simulink model "ES105A_StHlthSigNormn"  (R2013b)
settings: Solver=FixedStepDiscrete  SolverMode=SingleTasking  StartTime=0.0  StopTime=1  FixedStep=0.002  RelTol=1e-3
undefined symbols (not defined in the file): ARCHGLBPRM_FLOATZEROTHD_ULS_F32, CurrMeasCorrlnMaxErrCurr, CURRMOTSUMDIVBYZEROPROTNVAL_AMPR_F32, DIGTQDIVBYZEROPROTNVAL_HWNWTMTR_F32, DutyCycThermProtnDutyCycFildThd, EcuTMeasRngDiagcMax, EcuTMeasRngDiagcMin, EotLrngAuthyStrtLrn, FRICESTIMNDIVBYZEROPROTNVAL_HWNWTMTR_F32, HLTH0PERC_CNT_U08, HLTH100PERC_CNT_F32, HLTH100PERC_CNT_U08, HLTH50PERC_CNT_U08, HwTqCorrlnChATraSumSetFltThd, HwTqCorrlnChBTraSumSetFltThd, HWTQIDPTSIG_CNT_U08, MOTAG2MEAS_VALMAXERR_VOLTSQD_F32, MOTAG2MEAS_VALMINERR_VOLTSQD_F32, MOTAGCORRLN_MOTAGCORRLNERRTHD_MOTREVELEC_U0P16, MotDrvDiagcErrThd, MOTPOS2DIVBYZEROPROTNVAL2_VOLTSQD_F32, MOTPOS2DIVBYZEROPROTNVAL_VOLTSQD_F32, MOTPOSNERRDIVBYZEROPROTNVAL_MOTREV_U16, MOTPOSNERRZEROTHD_MOTREV_U0P16, NtcNr1, NtcSts1, PHAVLTGDIVBYZEROPROTNVAL_NANOSEC_F32, SigQlfr1, STHLTHSCAGFAC_CNT_F32, StHlthSigNormnAbsltMotPosDifStHlthDiagThd, StHlthSigNormnCurrMotSumStHlthDiagThd, StHlthSigNormnDigTqStHlthDiagThd, StHlthSigNormnDutyCycFltLimThd, StHlthSigNormnHiCtrlrT, StHlthSigNormnIdptSigStHlthSca, StHlthSigNormnLoCtrlrT, StHlthSigNormnMaxFricThd, StHlthSigNormnMinRackTrvlLim, StHlthSigNormnMotPosStHlthDiagThd, StHlthSigNormnMotVelCal, StHlthSigNormnPhaInfoStHlthDiagThd, StHlthSigNormnStHlthCorrlnErr, StHlthSigNormnStHlthCurrMotSum, StHlthSigNormnStHlthPhaInfo, StHlthSigNormnValMaxStHlthErr, StHlthSigNormnValMinStHlthErr, StHlthSigNormnWhlImbRejctnThd, SysGlbPrmMotPoleCnt, TSTHLTH0PERC_CNT_U08, u2, u3, u4, VLTGSTHLTH0PERC_CNT_U08
libraries: NxtrLim x39, simulink x33, NxtrAbslt x4
(part 6 of 10)

== system ES105A_StHlthSigNormn/StHlthSigNormn/UpdRawSig/Digital Torque Sensor /DigTqSnsrAStHlth Calc/If Action Subsystem1 ==
  HwTqChACorrlnTraErr : Inport
  Action Port : ActionPort  ActionType=else
  Abslt_f32_f32 : NxtrAbslt/Abslt_f32_f32  SFunctionSpec=single y1 = Abslt_f32_f32(single u1)
      settings: AttributesFormatString=%<Name>
  Constant2 : Constant  OutDataTypeStr=single
      settings: AttributesFormatString=%<OutDataTypeStr>
  Constant3 : Constant  Value=STHLTHSCAGFAC_CNT_F32
  CopyRight2 : Subsystem  Description=|  mask(Copyright Information){none=on}
      | Copyright info block.                                               
      |                                                                     
      | Place copyright information at the top of every subsystem in design.
      mask prompts: none "No parameters"
      mask help: Place copyright information at the top of every subsystem in design.
      mask Display:
      | NxtrConf = 'Nexteer Confidential';
      | 
      | sys = bdroot; %handle for the current model ("system")
      | first = get_param(sys,'Created');
      | first = first(end-3:end);  %year is last four digits
      | 
      | last = get_param(sys,'LastModifiedDate');
      | if isempty(last)
      |     last = datestr(now,'yyyy');
      | else
      |     last = last(end-3:end);
      | end
      | 
      | if strcmp(first,last)
      |     fprintf('%s -- Copyright %s Nexteer',NxtrConf,first)
      | else
      |     fprintf('%s -- %s%s- %s Nexteer',NxtrConf,char(169),first,last)
      | end
  Data Type Conversion : DataTypeConversion  OutDataTypeStr=uint8
  Devide by Zero Protection for Cal : Subsystem
  Divide : Product  Inputs=*/
  LimStat_f32 : NxtrLim/LimStat_f32  LoLim=STHLTHFLOATZEROVAL_ULS_F32  HiLim=STHLTHFLOATTWOFIFTYFIVEVAL_ULS_F32
      settings: AttributesFormatString=|
      | Low Limit: %<LoLim>
      | High Limit:%<HiLim>
  Product : Product
  Subtract : Sum  Inputs=+-
  DigTqSnsrAStHlth : Outport
  wires:
  HwTqChACorrlnTraErr/1 -> Divide/1
  Divide/1 -> Abslt_f32_f32/1
  Abslt_f32_f32/1 -> Subtract/2
  Constant2/1 -> Subtract/1
  Constant3/1 -> Product/2
  Data Type Conversion/1 -> DigTqSnsrAStHlth/1
  Subtract/1 -> Product/1
  Devide by Zero Protection for Cal/1(HwTqCorrlnChATraSumSetFltThd) -> Divide/2
  LimStat_f32/1 -> Data Type Conversion/1
  Product/1 -> LimStat_f32/1

== system ES105A_StHlthSigNormn/StHlthSigNormn/UpdRawSig/Digital Torque Sensor /DigTqSnsrBStHlth Calc/CopyRight2 ==

== system ES105A_StHlthSigNormn/StHlthSigNormn/UpdRawSig/Digital Torque Sensor /DigTqSnsrBStHlth Calc/If Action Subsystem2 ==
  Action Port : ActionPort  ActionType=then
  Constant : Constant  Value=HLTH0PERC_CNT_U08  OutDataTypeStr=uint8
  CopyRight2 : Subsystem  Description=|  mask(Copyright Information){none=on}
      | Copyright info block.                                               
      |                                                                     
      | Place copyright information at the top of every subsystem in design.
      mask prompts: none "No parameters"
      mask help: Place copyright information at the top of every subsystem in design.
      mask Display:
      | NxtrConf = 'Nexteer Confidential';
      | 
      | sys = bdroot; %handle for the current model ("system")
      | first = get_param(sys,'Created');
      | first = first(end-3:end);  %year is last four digits
      | 
      | last = get_param(sys,'LastModifiedDate');
      | if isempty(last)
      |     last = datestr(now,'yyyy');
      | else
      |     last = last(end-3:end);
      | end
      | 
      | if strcmp(first,last)
      |     fprintf('%s -- Copyright %s Nexteer',NxtrConf,first)
      | else
      |     fprintf('%s -- %s%s- %s Nexteer',NxtrConf,char(169),first,last)
      | end
  DigTqSnsrBStHlth : Outport
  wires:
  Constant/1 -> DigTqSnsrBStHlth/1

== system ES105A_StHlthSigNormn/StHlthSigNormn/UpdRawSig/Digital Torque Sensor /DigTqSnsrBStHlth Calc/If Action Subsystem3 ==
  HwTqChBCorrlnTraErr : Inport
  Action Port : ActionPort  ActionType=else
  Abslt_f32_f32 : NxtrAbslt/Abslt_f32_f32  SFunctionSpec=single y1 = Abslt_f32_f32(single u1)
      settings: AttributesFormatString=%<Name>
  Constant2 : Constant  OutDataTypeStr=single
      settings: AttributesFormatString=%<OutDataTypeStr>
  Constant3 : Constant  Value=STHLTHSCAGFAC_CNT_F32
  CopyRight2 : Subsystem  Description=|  mask(Copyright Information){none=on}
      | Copyright info block.                                               
      |                                                                     
      | Place copyright information at the top of every subsystem in design.
      mask prompts: none "No parameters"
      mask help: Place copyright information at the top of every subsystem in design.
      mask Display:
      | NxtrConf = 'Nexteer Confidential';
      | 
      | sys = bdroot; %handle for the current model ("system")
      | first = get_param(sys,'Created');
      | first = first(end-3:end);  %year is last four digits
      | 
      | last = get_param(sys,'LastModifiedDate');
      | if isempty(last)
      |     last = datestr(now,'yyyy');
      | else
      |     last = last(end-3:end);
      | end
      | 
      | if strcmp(first,last)
      |     fprintf('%s -- Copyright %s Nexteer',NxtrConf,first)
      | else
      |     fprintf('%s -- %s%s- %s Nexteer',NxtrConf,char(169),first,last)
      | end
  Data Type Conversion : DataTypeConversion  OutDataTypeStr=uint8
  Devide by Zero Protection for Cal : Subsystem
  Divide : Product  Inputs=*/
  LimStat_f32 : NxtrLim/LimStat_f32  LoLim=STHLTHFLOATZEROVAL_ULS_F32  HiLim=STHLTHFLOATTWOFIFTYFIVEVAL_ULS_F32
      settings: AttributesFormatString=|
      | Low Limit: %<LoLim>
      | High Limit:%<HiLim>
  Product : Product
  Subtract : Sum  Inputs=+-
  DigTqSnsrBStHlth : Outport
  wires:
  HwTqChBCorrlnTraErr/1 -> Divide/1
  Divide/1 -> Abslt_f32_f32/1
  Abslt_f32_f32/1 -> Subtract/2
  Constant2/1 -> Subtract/1
  Constant3/1 -> Product/2
  Subtract/1 -> Product/1
  Devide by Zero Protection for Cal/1(HwTqCorrlnChBTraSumSetFltThd) -> Divide/2
  LimStat_f32/1 -> Data Type Conversion/1
  Product/1 -> LimStat_f32/1
  Data Type Conversion/1 -> DigTqSnsrBStHlth/1

== system ES105A_StHlthSigNormn/StHlthSigNormn/UpdRawSig/Digital Torque Sensor /DigTqSnsrPhaStHlth/SetNtcSts ==
  note: Note:
      |
      | - "ISO Fault Debounce Design" Simulink block intent to use here for Simulation purpose only. Do not Code this block
  NtcNr : Inport
  NtcStInfo : Inport  Port=2
  NtcSts : Inport  Port=3
  DebStep : Inport  Port=4
  CopyRight2 : Subsystem  Description=|  mask(Copyright Information){none=on}
      | Copyright info block.                                               
      |                                                                     
      | Place copyright information at the top of every subsystem in design.
      mask prompts: none "No parameters"
      mask help: Place copyright information at the top of every subsystem in design.
      mask Display:
      | NxtrConf = 'Nexteer Confidential';
      | 
      | sys = bdroot; %handle for the current model ("system")
      | first = get_param(sys,'Created');
      | first = first(end-3:end);  %year is last four digits
      | 
      | last = get_param(sys,'LastModifiedDate');
      | if isempty(last)
      |     last = datestr(now,'yyyy');
      | else
      |     last = last(end-3:end);
      | end
      | 
      | if strcmp(first,last)
      |     fprintf('%s -- Copyright %s Nexteer',NxtrConf,first)
      | else
      |     fprintf('%s -- %s%s- %s Nexteer',NxtrConf,char(169),first,last)
      | end
  Data Store Write : DataStoreWrite  DataStoreName=NtcQlfr0X1D0
  Ground : Ground
  ISO Fault Debounce Design : Stateflow chart  TreatAsAtomicUnit=on
      settings: AttributesFormatString=|
      | Simulation Purpose Only.
      | Do Not Code this block
      | Diagnostic Manager Owns this requirement
  Terminator : Terminator
  Terminator1 : Terminator
  wires:
  NtcStInfo/1 -> Terminator1/1
  NtcNr/1 -> Terminator/1
  NtcSts/1 -> ISO Fault Debounce Design/1(NtcSts)
  DebStep/1 -> ISO Fault Debounce Design/2(DebStep)
  ISO Fault Debounce Design/1(Qualifier) -> Data Store Write/1
  Ground/1 -> ISO Fault Debounce Design/3(SvcClr)

== system ES105A_StHlthSigNormn/StHlthSigNormn/UpdRawSig/Digital Torque Sensor /NTC Sts Calculation/CopyRight2 ==

== system ES105A_StHlthSigNormn/StHlthSigNormn/UpdRawSig/Digital Torque Sensor /NTC Sts Calculation/NtcFaild ==
  Action Port : ActionPort  ActionType=then
  Constant2 : Constant  Value=NtcSts1.NTCSTS_FAILD  OutDataTypeStr=Enum: NtcSts1
  CopyRight2 : Subsystem  Description=|  mask(Copyright Information){none=on}
      | Copyright info block.                                               
      |                                                                     
      | Place copyright information at the top of every subsystem in design.
      mask prompts: none "No parameters"
      mask help: Place copyright information at the top of every subsystem in design.
      mask Display:
      | NxtrConf = 'Nexteer Confidential';
      | 
      | sys = bdroot; %handle for the current model ("system")
      | first = get_param(sys,'Created');
      | first = first(end-3:end);  %year is last four digits
      | 
      | last = get_param(sys,'LastModifiedDate');
      | if isempty(last)
      |     last = datestr(now,'yyyy');
      | else
      |     last = last(end-3:end);
      | end
      | 
      | if strcmp(first,last)
      |     fprintf('%s -- Copyright %s Nexteer',NxtrConf,first)
      | else
      |     fprintf('%s -- %s%s- %s Nexteer',NxtrConf,char(169),first,last)
      | end
  NtcFaild : Outport
  wires:
  Constant2/1 -> NtcFaild/1

== system ES105A_StHlthSigNormn/StHlthSigNormn/UpdRawSig/Digital Torque Sensor /NTC Sts Calculation/NtcPassd ==
  Action Port : ActionPort  ActionType=else
  Constant2 : Constant  Value=NtcSts1.NTCSTS_PASSD  OutDataTypeStr=Enum: NtcSts1
  CopyRight2 : Subsystem  Description=|  mask(Copyright Information){none=on}
      | Copyright info block.                                               
      |                                                                     
      | Place copyright information at the top of every subsystem in design.
      mask prompts: none "No parameters"
      mask help: Place copyright information at the top of every subsystem in design.
      mask Display:
      | NxtrConf = 'Nexteer Confidential';
      | 
      | sys = bdroot; %handle for the current model ("system")
      | first = get_param(sys,'Created');
      | first = first(end-3:end);  %year is last four digits
      | 
      | last = get_param(sys,'LastModifiedDate');
      | if isempty(last)
      |     last = datestr(now,'yyyy');
      | else
      |     last = last(end-3:end);
      | end
      | 
      | if strcmp(first,last)
      |     fprintf('%s -- Copyright %s Nexteer',NxtrConf,first)
      | else
      |     fprintf('%s -- %s%s- %s Nexteer',NxtrConf,char(169),first,last)
      | end
  NtcPassd : Outport
  wires:
  Constant2/1 -> NtcPassd/1

== system ES105A_StHlthSigNormn/StHlthSigNormn/UpdRawSig/Duty Cycle Exceeded/If Action Subsystem/CopyRight2 ==

== system ES105A_StHlthSigNormn/StHlthSigNormn/UpdRawSig/Duty Cycle Exceeded/If Action Subsystem1/CopyRight2 ==

== system ES105A_StHlthSigNormn/StHlthSigNormn/UpdRawSig/Duty Cycle Exceeded/If Action Subsystem2/CopyRight2 ==

== system ES105A_StHlthSigNormn/StHlthSigNormn/UpdRawSig/Friction Estimation/If Action Subsystem3/CopyRight2 ==

== system ES105A_StHlthSigNormn/StHlthSigNormn/UpdRawSig/Friction Estimation/If Action Subsystem4/CopyRight2 ==

== system ES105A_StHlthSigNormn/StHlthSigNormn/UpdRawSig/Friction Estimation/If Action Subsystem4/Divide by Zero Protection for Cal ==
  EOLFric : Inport
  Add1 : Sum  Inputs=+-
  Constant : Constant  Value=ARCHGLBPRM_FLOATZEROTHD_ULS_F32
  Constant2 : Constant  Value=StHlthSigNormnMaxFricThd
  CopyRight2 : Subsystem  Description=|  mask(Copyright Information){none=on}
      | Copyright info block.                                               
      |                                                                     
      | Place copyright information at the top of every subsystem in design.
      mask prompts: none "No parameters"
      mask help: Place copyright information at the top of every subsystem in design.
      mask Display:
      | NxtrConf = 'Nexteer Confidential';
      | 
      | sys = bdroot; %handle for the current model ("system")
      | first = get_param(sys,'Created');
      | first = first(end-3:end);  %year is last four digits
      | 
      | last = get_param(sys,'LastModifiedDate');
      | if isempty(last)
      |     last = datestr(now,'yyyy');
      | else
      |     last = last(end-3:end);
      | end
      | 
      | if strcmp(first,last)
      |     fprintf('%s -- Copyright %s Nexteer',NxtrConf,first)
      | else
      |     fprintf('%s -- %s%s- %s Nexteer',NxtrConf,char(169),first,last)
      | end
  If : If  IfExpression=u1
  If Zero : Subsystem  TreatAsAtomicUnit=on
  Merge : Merge
  Non Zero : Subsystem  TreatAsAtomicUnit=on
  Relational Operator : RelationalOperator  Operator=<=  OutDataTypeStr=boolean
  FricEstDelta : Outport
  wires:
  If/1 -> If Zero/Action
  If/2 -> Non Zero/Action
  If Zero/1(Out1) -> Merge/1
  Non Zero/1(Out1) -> Merge/2
  Merge/1 -> FricEstDelta/1
  Relational Operator/1 -> If/1
  Constant/1 -> Relational Operator/2
  Constant2/1 -> Add1/1
  EOLFric/1 -> Add1/2
  Add1/1 -> Non Zero/1(In1), Relational Operator/1

== system ES105A_StHlthSigNormn/StHlthSigNormn/UpdRawSig/Motor Position 2 /If Action Subsystem/CopyRight2 ==

== system ES105A_StHlthSigNormn/StHlthSigNormn/UpdRawSig/Motor Position 2 /If Action Subsystem/If Action Subsystem ==
  Action Port : ActionPort  ActionType=then
  Constant : Constant  Value=HLTH0PERC_CNT_U08
  CopyRight2 : Subsystem  Description=|  mask(Copyright Information){none=on}
      | Copyright info block.                                               
      |                                                                     
      | Place copyright information at the top of every subsystem in design.
      mask prompts: none "No parameters"
      mask help: Place copyright information at the top of every subsystem in design.
      mask Display:
      | NxtrConf = 'Nexteer Confidential';
      | 
      | sys = bdroot; %handle for the current model ("system")
      | first = get_param(sys,'Created');
      | first = first(end-3:end);  %year is last four digits
      | 
      | last = get_param(sys,'LastModifiedDate');
      | if isempty(last)
      |     last = datestr(now,'yyyy');
      | else
      |     last = last(end-3:end);
      | end
      | 
      | if strcmp(first,last)
      |     fprintf('%s -- Copyright %s Nexteer',NxtrConf,first)
      | else
      |     fprintf('%s -- %s%s- %s Nexteer',NxtrConf,char(169),first,last)
      | end
  MotPosStHlth : Outport
  wires:
  Constant/1 -> MotPosStHlth/1

== system ES105A_StHlthSigNormn/StHlthSigNormn/UpdRawSig/Motor Position 2 /If Action Subsystem/If Action Subsystem1 ==
  MotAg2VltgSqd : Inport
  Action Port : ActionPort  ActionType=elseif
  Constant : Constant  Value=MOTAG2MEAS_VALMINERR_VOLTSQD_F32
  Constant3 : Constant  Value=STHLTHSCAGFAC_CNT_F32
  CopyRight2 : Subsystem  Description=|  mask(Copyright Information){none=on}
      | Copyright info block.                                               
      |                                                                     
      | Place copyright information at the top of every subsystem in design.
      mask prompts: none "No parameters"
      mask help: Place copyright information at the top of every subsystem in design.
      mask Display:
      | NxtrConf = 'Nexteer Confidential';
      | 
      | sys = bdroot; %handle for the current model ("system")
      | first = get_param(sys,'Created');
      | first = first(end-3:end);  %year is last four digits
      | 
      | last = get_param(sys,'LastModifiedDate');
      | if isempty(last)
      |     last = datestr(now,'yyyy');
      | else
      |     last = last(end-3:end);
      | end
      | 
      | if strcmp(first,last)
      |     fprintf('%s -- Copyright %s Nexteer',NxtrConf,first)
      | else
      |     fprintf('%s -- %s%s- %s Nexteer',NxtrConf,char(169),first,last)
      | end
  Data Type Conversion : DataTypeConversion  OutDataTypeStr=uint8
  Divide : Product  Inputs=*/
  Divide by Zero Protection for Cal : Subsystem
  LimStat_f32 : NxtrLim/LimStat_f32  LoLim=STHLTHFLOATZEROVAL_ULS_F32  HiLim=STHLTHFLOATTWOFIFTYFIVEVAL_ULS_F32
      settings: AttributesFormatString=|
      | Low Limit: %<LoLim>
      | High Limit:%<HiLim>
  Product : Product
  Subtract : Sum  Inputs=+-
  MotPosStHlth : Outport
  wires:
  MotAg2VltgSqd/1 -> Subtract/1
  Constant/1 -> Subtract/2
  Subtract/1 -> Divide/1
  Constant3/1 -> Product/2
  Product/1 -> LimStat_f32/1
  Divide/1 -> Product/1
  Divide by Zero Protection for Cal/1(MotorPos2DeltaMin) -> Divide/2
  LimStat_f32/1 -> Data Type Conversion/1
  Data Type Conversion/1 -> MotPosStHlth/1

== system ES105A_StHlthSigNormn/StHlthSigNormn/UpdRawSig/Motor Position 2 /If Action Subsystem/If Action Subsystem2 ==
  MotAg2VltgSqd : Inport
  Action Port : ActionPort  ActionType=else
  Constant1 : Constant  Value=MOTAG2MEAS_VALMAXERR_VOLTSQD_F32
  Constant3 : Constant  Value=STHLTHSCAGFAC_CNT_F32
  CopyRight2 : Subsystem  Description=|  mask(Copyright Information){none=on}
      | Copyright info block.                                               
      |                                                                     
      | Place copyright information at the top of every subsystem in design.
      mask prompts: none "No parameters"
      mask help: Place copyright information at the top of every subsystem in design.
      mask Display:
      | NxtrConf = 'Nexteer Confidential';
      | 
      | sys = bdroot; %handle for the current model ("system")
      | first = get_param(sys,'Created');
      | first = first(end-3:end);  %year is last four digits
      | 
      | last = get_param(sys,'LastModifiedDate');
      | if isempty(last)
      |     last = datestr(now,'yyyy');
      | else
      |     last = last(end-3:end);
      | end
      | 
      | if strcmp(first,last)
      |     fprintf('%s -- Copyright %s Nexteer',NxtrConf,first)
      | else
      |     fprintf('%s -- %s%s- %s Nexteer',NxtrConf,char(169),first,last)
      | end
  Data Type Conversion : DataTypeConversion  OutDataTypeStr=uint8
  Divide : Product  Inputs=*/
  Divide by Zero Protection for Cal : Subsystem
  LimStat_f32 : NxtrLim/LimStat_f32  LoLim=STHLTHFLOATZEROVAL_ULS_F32  HiLim=STHLTHFLOATTWOFIFTYFIVEVAL_ULS_F32
      settings: AttributesFormatString=|
      | Low Limit: %<LoLim>
      | High Limit:%<HiLim>
  Product : Product
  Subtract1 : Sum  Inputs=+-
  MotPosStHlth : Outport
  wires:
  Constant3/1 -> Product/2
  Constant1/1 -> Subtract1/1
  MotAg2VltgSqd/1 -> Subtract1/2
  Subtract1/1 -> Divide/1
  Divide/1 -> Product/1
  Divide by Zero Protection for Cal/1(MotorPos2DeltaMax) -> Divide/2
  Product/1 -> LimStat_f32/1
  LimStat_f32/1 -> Data Type Conversion/1
  Data Type Conversion/1 -> MotPosStHlth/1

== system ES105A_StHlthSigNormn/StHlthSigNormn/UpdRawSig/Motor Position 2 /If Action Subsystem1/CopyRight2 ==

== system ES105A_StHlthSigNormn/StHlthSigNormn/UpdRawSig/Motor Position 2 /NTC Sts Calculation/CopyRight2 ==

== system ES105A_StHlthSigNormn/StHlthSigNormn/UpdRawSig/Motor Position 2 /NTC Sts Calculation/NtcFaild ==
  Action Port : ActionPort  ActionType=then
  Constant2 : Constant  Value=NtcSts1.NTCSTS_FAILD  OutDataTypeStr=Enum: NtcSts1
  CopyRight2 : Subsystem  Description=|  mask(Copyright Information){none=on}
      | Copyright info block.                                               
      |                                                                     
      | Place copyright information at the top of every subsystem in design.
      mask prompts: none "No parameters"
      mask help: Place copyright information at the top of every subsystem in design.
      mask Display:
      | NxtrConf = 'Nexteer Confidential';
      | 
      | sys = bdroot; %handle for the current model ("system")
      | first = get_param(sys,'Created');
      | first = first(end-3:end);  %year is last four digits
      | 
      | last = get_param(sys,'LastModifiedDate');
      | if isempty(last)
      |     last = datestr(now,'yyyy');
      | else
      |     last = last(end-3:end);
      | end
      | 
      | if strcmp(first,last)
      |     fprintf('%s -- Copyright %s Nexteer',NxtrConf,first)
      | else
      |     fprintf('%s -- %s%s- %s Nexteer',NxtrConf,char(169),first,last)
      | end
  NtcFaild : Outport
  wires:
  Constant2/1 -> NtcFaild/1

== system ES105A_StHlthSigNormn/StHlthSigNormn/UpdRawSig/Motor Position 2 /NTC Sts Calculation/NtcPassd ==
  Action Port : ActionPort  ActionType=else
  Constant2 : Constant  Value=NtcSts1.NTCSTS_PASSD  OutDataTypeStr=Enum: NtcSts1
  CopyRight2 : Subsystem  Description=|  mask(Copyright Information){none=on}
      | Copyright info block.                                               
      |                                                                     
      | Place copyright information at the top of every subsystem in design.
      mask prompts: none "No parameters"
      mask help: Place copyright information at the top of every subsystem in design.
      mask Display:
      | NxtrConf = 'Nexteer Confidential';
      | 
      | sys = bdroot; %handle for the current model ("system")
      | first = get_param(sys,'Created');
      | first = first(end-3:end);  %year is last four digits
      | 
      | last = get_param(sys,'LastModifiedDate');
      | if isempty(last)
      |     last = datestr(now,'yyyy');
      | else
      |     last = last(end-3:end);
      | end
      | 
      | if strcmp(first,last)
      |     fprintf('%s -- Copyright %s Nexteer',NxtrConf,first)
      | else
      |     fprintf('%s -- %s%s- %s Nexteer',NxtrConf,char(169),first,last)
      | end
  NtcPassd : Outport
  wires:
  Constant2/1 -> NtcPassd/1

== system ES105A_StHlthSigNormn/StHlthSigNormn/UpdRawSig/Motor Position 2 /NtcMotPosStHlth/SetNtcSts ==
  note: Note:
      |
      | - "ISO Fault Debounce Design" Simulink block intent to use here for Simulation purpose only. Do not Code this block
  NtcNr : Inport
  NtcStInfo : Inport  Port=2
  NtcSts : Inport  Port=3
  DebStep : Inport  Port=4
  CopyRight2 : Subsystem  Description=|  mask(Copyright Information){none=on}
      | Copyright info block.                                               
      |                                                                     
      | Place copyright information at the top of every subsystem in design.
      mask prompts: none "No parameters"
      mask help: Place copyright information at the top of every subsystem in design.
      mask Display:
      | NxtrConf = 'Nexteer Confidential';
      | 
      | sys = bdroot; %handle for the current model ("system")
      | first = get_param(sys,'Created');
      | first = first(end-3:end);  %year is last four digits
      | 
      | last = get_param(sys,'LastModifiedDate');
      | if isempty(last)
      |     last = datestr(now,'yyyy');
      | else
      |     last = last(end-3:end);
      | end
      | 
      | if strcmp(first,last)
      |     fprintf('%s -- Copyright %s Nexteer',NxtrConf,first)
      | else
      |     fprintf('%s -- %s%s- %s Nexteer',NxtrConf,char(169),first,last)
      | end
  Data Store Write : DataStoreWrite  DataStoreName=NtcQlfr0X1D1
  Ground : Ground
  ISO Fault Debounce Design : Stateflow chart  TreatAsAtomicUnit=on
      settings: AttributesFormatString=|
      | Simulation Purpose Only.
      | Do Not Code this block
      | Diagnostic Manager Owns this requirement
  Terminator : Terminator
  Terminator1 : Terminator
  wires:
  NtcStInfo/1 -> Terminator1/1
  NtcNr/1 -> Terminator/1
  NtcSts/1 -> ISO Fault Debounce Design/1(NtcSts)
  DebStep/1 -> ISO Fault Debounce Design/2(DebStep)
  ISO Fault Debounce Design/1(Qualifier) -> Data Store Write/1
  Ground/1 -> ISO Fault Debounce Design/3(SvcClr)

== system ES105A_StHlthSigNormn/StHlthSigNormn/UpdRawSig/Motor Position Error /AbsltMotPosABDifStHlth Calc/CopyRight2 ==

== system ES105A_StHlthSigNormn/StHlthSigNormn/UpdRawSig/Motor Position Error /AbsltMotPosABDifStHlth Calc/If Action Subsystem ==
  MotAgABErrTerm : Inport
  Action Port : ActionPort  ActionType=then
  CopyRight2 : Subsystem  Description=|  mask(Copyright Information){none=on}
      | Copyright info block.                                               
      |                                                                     
      | Place copyright information at the top of every subsystem in design.
      mask prompts: none "No parameters"
      mask help: Place copyright information at the top of every subsystem in design.
      mask Display:
      | NxtrConf = 'Nexteer Confidential';
      | 
      | sys = bdroot; %handle for the current model ("system")
      | first = get_param(sys,'Created');
      | first = first(end-3:end);  %year is last four digits
      | 
      | last = get_param(sys,'LastModifiedDate');
      | if isempty(last)
      |     last = datestr(now,'yyyy');
      | else
      |     last = last(end-3:end);
      | end
      | 
      | if strcmp(first,last)
      |     fprintf('%s -- Copyright %s Nexteer',NxtrConf,first)
      | else
      |     fprintf('%s -- %s%s- %s Nexteer',NxtrConf,char(169),first,last)
      | end
  Data Store Read : DataStoreRead  DataStoreName=MotAgCorrlnErrThd
  If : If  IfExpression=u1
  If Action Subsystem : Subsystem  TreatAsAtomicUnit=on
  If Action Subsystem1 : Subsystem  TreatAsAtomicUnit=on
  Merge : Merge
  Relational Operator : RelationalOperator  OutDataTypeStr=boolean
  AbsltMotPosABDiffStHlth : Outport
  wires:
  MotAgABErrTerm/1 -> Relational Operator/1, [MotAgABErrTerm]
  Data Store Read/1 -> Relational Operator/2
  Relational Operator/1 -> If/1
  If/1 -> If Action Subsystem/Action
  If/2 -> If Action Subsystem1/Action
  [MotAgABErrTerm] -> If Action Subsystem1/1(MotAgABErrTerm)
  If Action Subsystem/1(AbsltMotPosABDiffStHlth) -> Merge/1
  If Action Subsystem1/1(AbsltMotPosABDiffStHlth) -> Merge/2
  Merge/1 -> AbsltMotPosABDiffStHlth/1

== system ES105A_StHlthSigNormn/StHlthSigNormn/UpdRawSig/Motor Position Error /AbsltMotPosABDifStHlth Calc/If Action Subsystem1 ==
  Action Port : ActionPort  ActionType=else
  Constant : Constant  Value=HLTH100PERC_CNT_U08
  CopyRight2 : Subsystem  Description=|  mask(Copyright Information){none=on}
      | Copyright info block.                                               
      |                                                                     
      | Place copyright information at the top of every subsystem in design.
      mask prompts: none "No parameters"
      mask help: Place copyright information at the top of every subsystem in design.
      mask Display:
      | NxtrConf = 'Nexteer Confidential';
      | 
      | sys = bdroot; %handle for the current model ("system")
      | first = get_param(sys,'Created');
      | first = first(end-3:end);  %year is last four digits
      | 
      | last = get_param(sys,'LastModifiedDate');
      | if isempty(last)
      |     last = datestr(now,'yyyy');
      | else
      |     last = last(end-3:end);
      | end
      | 
      | if strcmp(first,last)
      |     fprintf('%s -- Copyright %s Nexteer',NxtrConf,first)
      | else
      |     fprintf('%s -- %s%s- %s Nexteer',NxtrConf,char(169),first,last)
      | end
  AbsltMotPosABDiffStHlth : Outport
  wires:
  Constant/1 -> AbsltMotPosABDiffStHlth/1

== system ES105A_StHlthSigNormn/StHlthSigNormn/UpdRawSig/Motor Position Error /AbsltMotPosACDifStHlth Calc/CopyRight2 ==

== system ES105A_StHlthSigNormn/StHlthSigNormn/UpdRawSig/Motor Position Error /AbsltMotPosACDifStHlth Calc/If Action Subsystem4 ==
  MotAgACErrTerm : Inport
  Action Port : ActionPort  ActionType=then
  CopyRight2 : Subsystem  Description=|  mask(Copyright Information){none=on}
      | Copyright info block.                                               
      |                                                                     
      | Place copyright information at the top of every subsystem in design.
      mask prompts: none "No parameters"
      mask help: Place copyright information at the top of every subsystem in design.
      mask Display:
      | NxtrConf = 'Nexteer Confidential';
      | 
      | sys = bdroot; %handle for the current model ("system")
      | first = get_param(sys,'Created');
      | first = first(end-3:end);  %year is last four digits
      | 
      | last = get_param(sys,'LastModifiedDate');
      | if isempty(last)
      |     last = datestr(now,'yyyy');
      | else
      |     last = last(end-3:end);
      | end
      | 
      | if strcmp(first,last)
      |     fprintf('%s -- Copyright %s Nexteer',NxtrConf,first)
      | else
      |     fprintf('%s -- %s%s- %s Nexteer',NxtrConf,char(169),first,last)
      | end
  Data Store Read : DataStoreRead  DataStoreName=MotAgCorrlnErrThd
  If : If  IfExpression=u1
  If Action Subsystem : Subsystem  TreatAsAtomicUnit=on
  If Action Subsystem1 : Subsystem  TreatAsAtomicUnit=on
  Merge : Merge
  Relational Operator : RelationalOperator  OutDataTypeStr=boolean
  AbsltMotPosACDiffStHlth : Outport
  wires:
  MotAgACErrTerm/1 -> [MotAgACErrTerm], Relational Operator/1
  Data Store Read/1 -> Relational Operator/2
  Relational Operator/1 -> If/1
  If/1 -> If Action Subsystem/Action
  If/2 -> If Action Subsystem1/Action
  [MotAgACErrTerm] -> If Action Subsystem1/1(MotAgACErrTerm)
  If Action Subsystem/1(AbsltMotPosACDiffStHlth) -> Merge/1
  If Action Subsystem1/1(AbsltMotPosACDiffStHlth) -> Merge/2
  Merge/1 -> AbsltMotPosACDiffStHlth/1

== system ES105A_StHlthSigNormn/StHlthSigNormn/UpdRawSig/Motor Position Error /AbsltMotPosACDifStHlth Calc/If Action Subsystem5 ==
  Action Port : ActionPort  ActionType=else
  Constant : Constant  Value=HLTH100PERC_CNT_U08
  CopyRight2 : Subsystem  Description=|  mask(Copyright Information){none=on}
      | Copyright info block.                                               
      |                                                                     
      | Place copyright information at the top of every subsystem in design.
      mask prompts: none "No parameters"
      mask help: Place copyright information at the top of every subsystem in design.
      mask Display:
      | NxtrConf = 'Nexteer Confidential';
      | 
      | sys = bdroot; %handle for the current model ("system")
      | first = get_param(sys,'Created');
      | first = first(end-3:end);  %year is last four digits
      | 
      | last = get_param(sys,'LastModifiedDate');
      | if isempty(last)
      |     last = datestr(now,'yyyy');
      | else
      |     last = last(end-3:end);
      | end
      | 
      | if strcmp(first,last)
      |     fprintf('%s -- Copyright %s Nexteer',NxtrConf,first)
      | else
      |     fprintf('%s -- %s%s- %s Nexteer',NxtrConf,char(169),first,last)
      | end
  AbsltMotPosACDiffStHlth : Outport
  wires:
  Constant/1 -> AbsltMotPosACDiffStHlth/1

== system ES105A_StHlthSigNormn/StHlthSigNormn/UpdRawSig/Motor Position Error /AbsltMotPosBCDifStHlth Calc/CopyRight2 ==

== system ES105A_StHlthSigNormn/StHlthSigNormn/UpdRawSig/Motor Position Error /AbsltMotPosBCDifStHlth Calc/If Action Subsystem8 ==
  MotAgBCErrTerm : Inport
  Action Port : ActionPort  ActionType=then
  CopyRight2 : Subsystem  Description=|  mask(Copyright Information){none=on}
      | Copyright info block.                                               
      |                                                                     
      | Place copyright information at the top of every subsystem in design.
      mask prompts: none "No parameters"
      mask help: Place copyright information at the top of every subsystem in design.
      mask Display:
      | NxtrConf = 'Nexteer Confidential';
      | 
      | sys = bdroot; %handle for the current model ("system")
      | first = get_param(sys,'Created');
      | first = first(end-3:end);  %year is last four digits
      | 
      | last = get_param(sys,'LastModifiedDate');
      | if isempty(last)
      |     last = datestr(now,'yyyy');
      | else
      |     last = last(end-3:end);
      | end
      | 
      | if strcmp(first,last)
      |     fprintf('%s -- Copyright %s Nexteer',NxtrConf,first)
      | else
      |     fprintf('%s -- %s%s- %s Nexteer',NxtrConf,char(169),first,last)
      | end
  Data Store Read : DataStoreRead  DataStoreName=MotAgCorrlnErrThd
  If : If  IfExpression=u1
  If Action Subsystem : Subsystem  TreatAsAtomicUnit=on
  If Action Subsystem1 : Subsystem  TreatAsAtomicUnit=on
  Merge : Merge
  Relational Operator : RelationalOperator  OutDataTypeStr=boolean
  AbsltMotPosBCDiffStHlth : Outport
  wires:
  MotAgBCErrTerm/1 -> [MotAgBCErrTerm], Relational Operator/1
  Data Store Read/1 -> Relational Operator/2
  Relational Operator/1 -> If/1
  If/1 -> If Action Subsystem/Action
  If/2 -> If Action Subsystem1/Action
  [MotAgBCErrTerm] -> If Action Subsystem1/1(MotAgBCErrTerm)
  If Action Subsystem/1(AbsltMotPosBCDiffStHlth) -> Merge/1
  If Action Subsystem1/1(AbsltMotPosBCDiffStHlth) -> Merge/2
  Merge/1 -> AbsltMotPosBCDiffStHlth/1

== system ES105A_StHlthSigNormn/StHlthSigNormn/UpdRawSig/Motor Position Error /AbsltMotPosBCDifStHlth Calc/If Action Subsystem9 ==
  Action Port : ActionPort  ActionType=else
  Constant : Constant  Value=HLTH100PERC_CNT_U08
  CopyRight2 : Subsystem  Description=|  mask(Copyright Information){none=on}
      | Copyright info block.                                               
      |                                                                     
      | Place copyright information at the top of every subsystem in design.
      mask prompts: none "No parameters"
      mask help: Place copyright information at the top of every subsystem in design.
      mask Display:
      | NxtrConf = 'Nexteer Confidential';
      | 
      | sys = bdroot; %handle for the current model ("system")
      | first = get_param(sys,'Created');
      | first = first(end-3:end);  %year is last four digits
      | 
      | last = get_param(sys,'LastModifiedDate');
      | if isempty(last)
      |     last = datestr(now,'yyyy');
      | else
      |     last = last(end-3:end);
      | end
      | 
      | if strcmp(first,last)
      |     fprintf('%s -- Copyright %s Nexteer',NxtrConf,first)
      | else
      |     fprintf('%s -- %s%s- %s Nexteer',NxtrConf,char(169),first,last)
      | end
  AbsMotPosBCDiffStHlth : Outport
  wires:
  Constant/1 -> AbsMotPosBCDiffStHlth/1

== system ES105A_StHlthSigNormn/StHlthSigNormn/UpdRawSig/Motor Position Error /AbsltMotPosPhaDifStHlth/SetNtcSts ==
  note: Note:
      |
      | - "ISO Fault Debounce Design" Simulink block intent to use here for Simulation purpose only. Do not Code this block
  NtcNr : Inport
  NtcStInfo : Inport  Port=2
  NtcSts : Inport  Port=3
  DebStep : Inport  Port=4
  CopyRight2 : Subsystem  Description=|  mask(Copyright Information){none=on}
      | Copyright info block.                                               
      |                                                                     
      | Place copyright information at the top of every subsystem in design.
      mask prompts: none "No parameters"
      mask help: Place copyright information at the top of every subsystem in design.
      mask Display:
      | NxtrConf = 'Nexteer Confidential';
      | 
      | sys = bdroot; %handle for the current model ("system")
      | first = get_param(sys,'Created');
      | first = first(end-3:end);  %year is last four digits
      | 
      | last = get_param(sys,'LastModifiedDate');
      | if isempty(last)
      |     last = datestr(now,'yyyy');
      | else
      |     last = last(end-3:end);
      | end
      | 
      | if strcmp(first,last)
      |     fprintf('%s -- Copyright %s Nexteer',NxtrConf,first)
      | else
      |     fprintf('%s -- %s%s- %s Nexteer',NxtrConf,char(169),first,last)
      | end
  Data Store Write : DataStoreWrite  DataStoreName=NtcQlfr0X1D2
  Ground : Ground
  ISO Fault Debounce Design : Stateflow chart  TreatAsAtomicUnit=on
      settings: AttributesFormatString=|
      | Simulation Purpose Only.
      | Do Not Code this block
      | Diagnostic Manager Owns this requirement
  Terminator : Terminator
  Terminator1 : Terminator
  wires:
  NtcStInfo/1 -> Terminator1/1
  NtcNr/1 -> Terminator/1
  NtcSts/1 -> ISO Fault Debounce Design/1(NtcSts)
  DebStep/1 -> ISO Fault Debounce Design/2(DebStep)
  ISO Fault Debounce Design/1(Qualifier) -> Data Store Write/1
  Ground/1 -> ISO Fault Debounce Design/3(SvcClr)

== system ES105A_StHlthSigNormn/StHlthSigNormn/UpdRawSig/Motor Position Error /NTC Sts Calculation/CopyRight2 ==

== system ES105A_StHlthSigNormn/StHlthSigNormn/UpdRawSig/Motor Position Error /NTC Sts Calculation/NtcFaild ==
  Action Port : ActionPort  ActionType=then
  Constant2 : Constant  Value=NtcSts1.NTCSTS_FAILD  OutDataTypeStr=Enum: NtcSts1
  CopyRight2 : Subsystem  Description=|  mask(Copyright Information){none=on}
      | Copyright info block.                                               
      |                                                                     
      | Place copyright information at the top of every subsystem in design.
      mask prompts: none "No parameters"
      mask help: Place copyright information at the top of every subsystem in design.
      mask Display:
      | NxtrConf = 'Nexteer Confidential';
      | 
      | sys = bdroot; %handle for the current model ("system")
      | first = get_param(sys,'Created');
      | first = first(end-3:end);  %year is last four digits
      | 
      | last = get_param(sys,'LastModifiedDate');
      | if isempty(last)
      |     last = datestr(now,'yyyy');
      | else
      |     last = last(end-3:end);
      | end
      | 
      | if strcmp(first,last)
      |     fprintf('%s -- Copyright %s Nexteer',NxtrConf,first)
      | else
      |     fprintf('%s -- %s%s- %s Nexteer',NxtrConf,char(169),first,last)
      | end
  NtcFaild : Outport
  wires:
  Constant2/1 -> NtcFaild/1

== system ES105A_StHlthSigNormn/StHlthSigNormn/UpdRawSig/Motor Position Error /NTC Sts Calculation/NtcPassd ==
  Action Port : ActionPort  ActionType=else
  Constant2 : Constant  Value=NtcSts1.NTCSTS_PASSD  OutDataTypeStr=Enum: NtcSts1
  CopyRight2 : Subsystem  Description=|  mask(Copyright Information){none=on}
      | Copyright info block.                                               
      |                                                                     
      | Place copyright information at the top of every subsystem in design.
      mask prompts: none "No parameters"
      mask help: Place copyright information at the top of every subsystem in design.
      mask Display:
      | NxtrConf = 'Nexteer Confidential';
      | 
      | sys = bdroot; %handle for the current model ("system")
      | first = get_param(sys,'Created');
      | first = first(end-3:end);  %year is last four digits
      | 
      | last = get_param(sys,'LastModifiedDate');
      | if isempty(last)
      |     last = datestr(now,'yyyy');
      | else
      |     last = last(end-3:end);
      | end
      | 
      | if strcmp(first,last)
      |     fprintf('%s -- Copyright %s Nexteer',NxtrConf,first)
      | else
      |     fprintf('%s -- %s%s- %s Nexteer',NxtrConf,char(169),first,last)
      | end
  NtcPassd : Outport
  wires:
  Constant2/1 -> NtcPassd/1

== system ES105A_StHlthSigNormn/StHlthSigNormn/UpdRawSig/Phase Voltage Verification/NTC Sts Calculation/CopyRight2 ==

== system ES105A_StHlthSigNormn/StHlthSigNormn/UpdRawSig/Phase Voltage Verification/NTC Sts Calculation/NtcFaild ==
  Action Port : ActionPort  ActionType=then
  Constant2 : Constant  Value=NtcSts1.NTCSTS_FAILD  OutDataTypeStr=Enum: NtcSts1
  CopyRight2 : Subsystem  Description=|  mask(Copyright Information){none=on}
      | Copyright info block.                                               
      |                                                                     
      | Place copyright information at the top of every subsystem in design.
      mask prompts: none "No parameters"
      mask help: Place copyright information at the top of every subsystem in design.
      mask Display:
      | NxtrConf = 'Nexteer Confidential';
      | 
      | sys = bdroot; %handle for the current model ("system")
      | first = get_param(sys,'Created');
      | first = first(end-3:end);  %year is last four digits
      | 
      | last = get_param(sys,'LastModifiedDate');
      | if isempty(last)
      |     last = datestr(now,'yyyy');
      | else
      |     last = last(end-3:end);
      | end
      | 
      | if strcmp(first,last)
      |     fprintf('%s -- Copyright %s Nexteer',NxtrConf,first)
      | else
      |     fprintf('%s -- %s%s- %s Nexteer',NxtrConf,char(169),first,last)
      | end
  NtcFaild : Outport
  wires:
  Constant2/1 -> NtcFaild/1

== system ES105A_StHlthSigNormn/StHlthSigNormn/UpdRawSig/Phase Voltage Verification/NTC Sts Calculation/NtcPassd ==
  Action Port : ActionPort  ActionType=else
  Constant2 : Constant  Value=NtcSts1.NTCSTS_PASSD  OutDataTypeStr=Enum: NtcSts1
  CopyRight2 : Subsystem  Description=|  mask(Copyright Information){none=on}
      | Copyright info block.                                               
      |                                                                     
      | Place copyright information at the top of every subsystem in design.
      mask prompts: none "No parameters"
      mask help: Place copyright information at the top of every subsystem in design.
      mask Display:
      | NxtrConf = 'Nexteer Confidential';
      | 
      | sys = bdroot; %handle for the current model ("system")
      | first = get_param(sys,'Created');
      | first = first(end-3:end);  %year is last four digits
      | 
      | last = get_param(sys,'LastModifiedDate');
      | if isempty(last)
      |     last = datestr(now,'yyyy');
      | else
      |     last = last(end-3:end);
      | end
      | 
      | if strcmp(first,last)
      |     fprintf('%s -- Copyright %s Nexteer',NxtrConf,first)
      | else
      |     fprintf('%s -- %s%s- %s Nexteer',NxtrConf,char(169),first,last)
      | end
  NtcPassd : Outport
  wires:
  Constant2/1 -> NtcPassd/1

== system ES105A_StHlthSigNormn/StHlthSigNormn/UpdRawSig/Phase Voltage Verification/PhaAStHlth Calc/CopyRight2 ==

== system ES105A_StHlthSigNormn/StHlthSigNormn/UpdRawSig/Phase Voltage Verification/PhaAStHlth Calc/If Action Subsystem ==
  MotDrvErrA : Inport
  Action Port : ActionPort  ActionType=then
  Constant : Constant  Value=MotDrvDiagcErrThd
  CopyRight2 : Subsystem  Description=|  mask(Copyright Information){none=on}
      | Copyright info block.                                               
      |                                                                     
      | Place copyright information at the top of every subsystem in design.
      mask prompts: none "No parameters"
      mask help: Place copyright information at the top of every subsystem in design.
      mask Display:
      | NxtrConf = 'Nexteer Confidential';
      | 
      | sys = bdroot; %handle for the current model ("system")
      | first = get_param(sys,'Created');
      | first = first(end-3:end);  %year is last four digits
      | 
      | last = get_param(sys,'LastModifiedDate');
      | if isempty(last)
      |     last = datestr(now,'yyyy');
      | else
      |     last = last(end-3:end);
      | end
      | 
      | if strcmp(first,last)
      |     fprintf('%s -- Copyright %s Nexteer',NxtrConf,first)
      | else
      |     fprintf('%s -- %s%s- %s Nexteer',NxtrConf,char(169),first,last)
      | end
  If : If  IfExpression=u1
  If Action Subsystem : Subsystem  TreatAsAtomicUnit=on
  If Action Subsystem1 : Subsystem  TreatAsAtomicUnit=on
  Merge : Merge
  Relational Operator : RelationalOperator  OutDataTypeStr=boolean
  PhaseAStHlth : Outport
  wires:
  MotDrvErrA/1 -> [MotDrvErrA], Relational Operator/1
  Constant/1 -> Relational Operator/2
  Relational Operator/1 -> If/1
  If/1 -> If Action Subsystem/Action
  If/2 -> If Action Subsystem1/Action
  [MotDrvErrA] -> If Action Subsystem1/1(MotDrvErrA)
  If Action Subsystem/1(PhaseAStHlth) -> Merge/1
  If Action Subsystem1/1(PhaseAStHlth) -> Merge/2
  Merge/1 -> PhaseAStHlth/1

== system ES105A_StHlthSigNormn/StHlthSigNormn/UpdRawSig/Phase Voltage Verification/PhaAStHlth Calc/If Action Subsystem1 ==
  Action Port : ActionPort  ActionType=else
  Constant : Constant  Value=HLTH100PERC_CNT_U08
  CopyRight2 : Subsystem  Description=|  mask(Copyright Information){none=on}
      | Copyright info block.                                               
      |                                                                     
      | Place copyright information at the top of every subsystem in design.
      mask prompts: none "No parameters"
      mask help: Place copyright information at the top of every subsystem in design.
      mask Display:
      | NxtrConf = 'Nexteer Confidential';
      | 
      | sys = bdroot; %handle for the current model ("system")
      | first = get_param(sys,'Created');
      | first = first(end-3:end);  %year is last four digits
      | 
      | last = get_param(sys,'LastModifiedDate');
      | if isempty(last)
      |     last = datestr(now,'yyyy');
      | else
      |     last = last(end-3:end);
      | end
      | 
      | if strcmp(first,last)
      |     fprintf('%s -- Copyright %s Nexteer',NxtrConf,first)
      | else
      |     fprintf('%s -- %s%s- %s Nexteer',NxtrConf,char(169),first,last)
      | end
  PhaseAStHlth : Outport
  wires:
  Constant/1 -> PhaseAStHlth/1

== system ES105A_StHlthSigNormn/StHlthSigNormn/UpdRawSig/Phase Voltage Verification/PhaBStHlth Calc/CopyRight2 ==

== system ES105A_StHlthSigNormn/StHlthSigNormn/UpdRawSig/Phase Voltage Verification/PhaBStHlth Calc/If Action Subsystem4 ==
  MotDrvErrB : Inport
  Action Port : ActionPort  ActionType=then
  Constant : Constant  Value=MotDrvDiagcErrThd
  CopyRight2 : Subsystem  Description=|  mask(Copyright Information){none=on}
      | Copyright info block.                                               
      |                                                                     
      | Place copyright information at the top of every subsystem in design.
      mask prompts: none "No parameters"
      mask help: Place copyright information at the top of every subsystem in design.
      mask Display:
      | NxtrConf = 'Nexteer Confidential';
      | 
      | sys = bdroot; %handle for the current model ("system")
      | first = get_param(sys,'Created');
      | first = first(end-3:end);  %year is last four digits
      | 
      | last = get_param(sys,'LastModifiedDate');
      | if isempty(last)
      |     last = datestr(now,'yyyy');
      | else
      |     last = last(end-3:end);
      | end
      | 
      | if strcmp(first,last)
      |     fprintf('%s -- Copyright %s Nexteer',NxtrConf,first)
      | else
      |     fprintf('%s -- %s%s- %s Nexteer',NxtrConf,char(169),first,last)
      | end
  If : If  IfExpression=u1
  If Action Subsystem : Subsystem  TreatAsAtomicUnit=on
  If Action Subsystem1 : Subsystem  TreatAsAtomicUnit=on
  Merge : Merge
  Relational Operator : RelationalOperator  OutDataTypeStr=boolean
  PhaseBStHlth : Outport
  wires:
  MotDrvErrB/1 -> [MotDrvErrB], Relational Operator/1
  Constant/1 -> Relational Operator/2
  Relational Operator/1 -> If/1
  If/1 -> If Action Subsystem/Action
  If/2 -> If Action Subsystem1/Action
  [MotDrvErrB] -> If Action Subsystem1/1(MotDrvErrB)
  If Action Subsystem/1(PhaseBStHlth) -> Merge/1
  If Action Subsystem1/1(PhaseBStHlth) -> Merge/2
  Merge/1 -> PhaseBStHlth/1
